simulink model "suspension_controller_road_condition2"  (R2020a)
settings: Solver=VariableStepAuto  StartTime=0.0  StopTime=10.0  MaxStep=0.1  RelTol=1e-3
values from neighbouring files (symbols this model uses):
  cfs = 1290    [half_car_parameter.m]
  cft = 1000    [half_car_parameter.m]
  crs = 1620    [half_car_parameter.m]
  crt = 1000    [half_car_parameter.m]
  iyy = 2460    [half_car_parameter.m]
  kfs = 19960    [half_car_parameter.m]
  kft = 175500    [half_car_parameter.m]
  krs = 17500    [half_car_parameter.m]
  krt = 175500    [half_car_parameter.m]
  lf = 2.3    [half_car_parameter.m]
  lr = 2.3    [half_car_parameter.m]
  mc = 700    [half_car_parameter.m]
  mf = 40    [half_car_parameter.m]
  mr = 35.5    [half_car_parameter.m]
(part 2 of 2)

== system suspension_controller_road_condition2/skyhook/body_sum/sky hook control ==
  zc_dot : Inport
  zc_dot - zf_dot : Inport  Port=2
  Constant : Constant  Value=2838
  Constant1 : Constant  Value=258
  If : If  IfExpression=u1 >= 0  ZeroCross=off
  If Action Subsystem : Subsystem  TreatAsAtomicUnit=on
  If Action Subsystem1 : Subsystem  TreatAsAtomicUnit=on
  Merge : Merge
  Product : Product
  Csa : Outport
  wires:
  zc_dot/1 -> Product/1
  Product/1 -> If/1
  If/1 -> If Action Subsystem/Action
  Constant/1 -> If Action Subsystem/1(In1)
  If/2 -> If Action Subsystem1/Action
  If Action Subsystem/1(Csa) -> Merge/1
  If Action Subsystem1/1(Out1) -> Merge/2
  Merge/1 -> Csa/1
  Constant1/1 -> If Action Subsystem1/1(In1)
  zc_dot - zf_dot/1 -> Product/2

== system suspension_controller_road_condition2/skyhook/body_sum/sky hook control1 ==
  zc_dot : Inport
  zc_dot - zr_dot : Inport  Port=2
  Constant : Constant  Value=2838
  Constant1 : Constant  Value=258
  If : If  IfExpression=u1 >= 0  ZeroCross=off
  If Action Subsystem : Subsystem  TreatAsAtomicUnit=on
  If Action Subsystem1 : Subsystem  TreatAsAtomicUnit=on
  Merge : Merge
  Product : Product
  Csa : Outport
  wires:
  zc_dot/1 -> Product/1
  Product/1 -> If/1
  If/1 -> If Action Subsystem/Action
  Constant/1 -> If Action Subsystem/1(In1)
  If/2 -> If Action Subsystem1/Action
  If Action Subsystem/1(Csa) -> Merge/1
  If Action Subsystem1/1(Out1) -> Merge/2
  Merge/1 -> Csa/1
  Constant1/1 -> If Action Subsystem1/1(In1)
  zc_dot - zr_dot/1 -> Product/2

== system suspension_controller_road_condition2/skyhook/front_sum/Road Condition2 ==
  Product : Product  Inputs=3
  Saturation : Saturate  LowerLimit=0
  Scope : Scope
  Signal Generator : SignalGenerator  Amplitude=0.15  Frequency=1.852
  Step : Step  SampleTime=1.08
  Step1 : Step  Before=1  After=0  SampleTime=4
  Output : Outport
  wires:
  Signal Generator/1 -> Product/1
  Step/1 -> Product/2
  Step1/1 -> Product/3
  Product/1 -> Output/1, Saturation/1
  Saturation/1 -> Scope/1

== system suspension_controller_road_condition2/skyhook/front_sum/sky hook control ==
  zc_dot : Inport
  zc_dot - zf_dot : Inport  Port=2
  Constant : Constant  Value=2838
  Constant1 : Constant  Value=258
  If : If  IfExpression=u1 >= 0  ZeroCross=off
  If Action Subsystem : Subsystem  TreatAsAtomicUnit=on
  If Action Subsystem1 : Subsystem  TreatAsAtomicUnit=on
  Merge : Merge
  Product : Product
  Csa : Outport
  wires:
  zc_dot/1 -> Product/1
  Product/1 -> If/1
  If/1 -> If Action Subsystem/Action
  Constant/1 -> If Action Subsystem/1(In1)
  If/2 -> If Action Subsystem1/Action
  If Action Subsystem/1(Csa) -> Merge/1
  If Action Subsystem1/1(Out1) -> Merge/2
  Merge/1 -> Csa/1
  Constant1/1 -> If Action Subsystem1/1(In1)
  zc_dot - zf_dot/1 -> Product/2

== system suspension_controller_road_condition2/skyhook/rear_sum/Road Condition2 ==
  Product : Product  Inputs=3
  Saturation : Saturate  LowerLimit=0
  Scope : Scope
  Signal Generator : SignalGenerator  Amplitude=0.15  Frequency=1.852
  Step : Step  SampleTime=1.08
  Step1 : Step  Before=1  After=0  SampleTime=4
  Output : Outport
  wires:
  Signal Generator/1 -> Product/1
  Step/1 -> Product/2
  Step1/1 -> Product/3
  Product/1 -> Output/1, Saturation/1
  Saturation/1 -> Scope/1

== system suspension_controller_road_condition2/skyhook/rear_sum/sky hook control ==
  zc_dot : Inport
  zc_dot - zr_dot : Inport  Port=2
  Constant : Constant  Value=2838
  Constant1 : Constant  Value=258
  If : If  IfExpression=u1 >= 0  ZeroCross=off
  If Action Subsystem : Subsystem  TreatAsAtomicUnit=on
  If Action Subsystem1 : Subsystem  TreatAsAtomicUnit=on
  Merge : Merge
  Product : Product
  Csa : Outport
  wires:
  zc_dot/1 -> Product/1
  Product/1 -> If/1
  If/1 -> If Action Subsystem/Action
  Constant/1 -> If Action Subsystem/1(In1)
  If/2 -> If Action Subsystem1/Action
  If Action Subsystem/1(Csa) -> Merge/1
  If Action Subsystem1/1(Out1) -> Merge/2
  Merge/1 -> Csa/1
  Constant1/1 -> If Action Subsystem1/1(In1)
  zc_dot - zr_dot/1 -> Product/2

== system suspension_controller_road_condition2/ground hook/body_sum/Ground hook control/If Action Subsystem ==
  In1 : Inport
  Action Port : ActionPort  ActionPortLabel=if(u1 >= 0)
  Csa : Outport
  wires:
  In1/1 -> Csa/1

== system suspension_controller_road_condition2/ground hook/body_sum/Ground hook control/If Action Subsystem1 ==
  In1 : Inport
  Action Port : ActionPort  ActionPortLabel=else
  Out1 : Outport
  wires:
  In1/1 -> Out1/1

== system suspension_controller_road_condition2/ground hook/body_sum/Ground hook control1/If Action Subsystem ==
  In1 : Inport
  Action Port : ActionPort  ActionPortLabel=if(u1 >= 0)
  Csa : Outport
  wires:
  In1/1 -> Csa/1

== system suspension_controller_road_condition2/ground hook/body_sum/Ground hook control1/If Action Subsystem1 ==
  In1 : Inport
  Action Port : ActionPort  ActionPortLabel=else
  Out1 : Outport
  wires:
  In1/1 -> Out1/1

== system suspension_controller_road_condition2/ground hook/front_sum/Ground hook control/If Action Subsystem ==
  In1 : Inport
  Action Port : ActionPort  ActionPortLabel=if(u1 >= 0)
  Csa : Outport
  wires:
  In1/1 -> Csa/1

== system suspension_controller_road_condition2/ground hook/front_sum/Ground hook control/If Action Subsystem1 ==
  In1 : Inport
  Action Port : ActionPort  ActionPortLabel=else
  Out1 : Outport
  wires:
  In1/1 -> Out1/1

== system suspension_controller_road_condition2/ground hook/rear_sum/Ground hook control1/If Action Subsystem ==
  In1 : Inport
  Action Port : ActionPort  ActionPortLabel=if(u1 >= 0)
  Csa : Outport
  wires:
  In1/1 -> Csa/1

== system suspension_controller_road_condition2/ground hook/rear_sum/Ground hook control1/If Action Subsystem1 ==
  In1 : Inport
  Action Port : ActionPort  ActionPortLabel=else
  Out1 : Outport
  wires:
  In1/1 -> Out1/1

== system suspension_controller_road_condition2/hybrid hook/body_sum/Hybrid controller/If Action Subsystem ==
  In1 : Inport
  Action Port : ActionPort  ActionPortLabel=if(u1 >= 0)
  Csa : Outport
  wires:
  In1/1 -> Csa/1

== system suspension_controller_road_condition2/hybrid hook/body_sum/Hybrid controller/If Action Subsystem1 ==
  In1 : Inport
  Action Port : ActionPort  ActionPortLabel=else
  Out1 : Outport
  wires:
  In1/1 -> Out1/1

== system suspension_controller_road_condition2/hybrid hook/body_sum/Hybrid controller/If Action Subsystem2 ==
  In1 : Inport
  Action Port : ActionPort  ActionPortLabel=if(u1 >= 0)
  Csa : Outport
  wires:
  In1/1 -> Csa/1

== system suspension_controller_road_condition2/hybrid hook/body_sum/Hybrid controller/If Action Subsystem3 ==
  In1 : Inport
  Action Port : ActionPort  ActionPortLabel=else
  Out1 : Outport
  wires:
  In1/1 -> Out1/1

== system suspension_controller_road_condition2/hybrid hook/body_sum/Hybrid controller1/If Action Subsystem ==
  In1 : Inport
  Action Port : ActionPort  ActionPortLabel=if(u1 >= 0)
  Csa : Outport
  wires:
  In1/1 -> Csa/1

== system suspension_controller_road_condition2/hybrid hook/body_sum/Hybrid controller1/If Action Subsystem1 ==
  In1 : Inport
  Action Port : ActionPort  ActionPortLabel=else
  Out1 : Outport
  wires:
  In1/1 -> Out1/1

== system suspension_controller_road_condition2/hybrid hook/body_sum/Hybrid controller1/If Action Subsystem2 ==
  In1 : Inport
  Action Port : ActionPort  ActionPortLabel=if(u1 >= 0)
  Csa : Outport
  wires:
  In1/1 -> Csa/1

== system suspension_controller_road_condition2/hybrid hook/body_sum/Hybrid controller1/If Action Subsystem3 ==
  In1 : Inport
  Action Port : ActionPort  ActionPortLabel=else
  Out1 : Outport
  wires:
  In1/1 -> Out1/1

== system suspension_controller_road_condition2/hybrid hook/front_sum/Hybrid controller/If Action Subsystem ==
  In1 : Inport
  Action Port : ActionPort  ActionPortLabel=if(u1 >= 0)
  Csa : Outport
  wires:
  In1/1 -> Csa/1

== system suspension_controller_road_condition2/hybrid hook/front_sum/Hybrid controller/If Action Subsystem1 ==
  In1 : Inport
  Action Port : ActionPort  ActionPortLabel=else
  Out1 : Outport
  wires:
  In1/1 -> Out1/1

== system suspension_controller_road_condition2/hybrid hook/front_sum/Hybrid controller/If Action Subsystem2 ==
  In1 : Inport
  Action Port : ActionPort  ActionPortLabel=if(u1 >= 0)
  Csa : Outport
  wires:
  In1/1 -> Csa/1

== system suspension_controller_road_condition2/hybrid hook/front_sum/Hybrid controller/If Action Subsystem3 ==
  In1 : Inport
  Action Port : ActionPort  ActionPortLabel=else
  Out1 : Outport
  wires:
  In1/1 -> Out1/1

== system suspension_controller_road_condition2/hybrid hook/rear_sum/Hybrid controller1/If Action Subsystem ==
  In1 : Inport
  Action Port : ActionPort  ActionPortLabel=if(u1 >= 0)
  Csa : Outport
  wires:
  In1/1 -> Csa/1

== system suspension_controller_road_condition2/hybrid hook/rear_sum/Hybrid controller1/If Action Subsystem1 ==
  In1 : Inport
  Action Port : ActionPort  ActionPortLabel=else
  Out1 : Outport
  wires:
  In1/1 -> Out1/1

== system suspension_controller_road_condition2/hybrid hook/rear_sum/Hybrid controller1/If Action Subsystem2 ==
  In1 : Inport
  Action Port : ActionPort  ActionPortLabel=if(u1 >= 0)
  Csa : Outport
  wires:
  In1/1 -> Csa/1

== system suspension_controller_road_condition2/hybrid hook/rear_sum/Hybrid controller1/If Action Subsystem3 ==
  In1 : Inport
  Action Port : ActionPort  ActionPortLabel=else
  Out1 : Outport
  wires:
  In1/1 -> Out1/1

== system suspension_controller_road_condition2/skyhook/body_sum/sky hook control/If Action Subsystem ==
  In1 : Inport
  Action Port : ActionPort  ActionPortLabel=if(u1 >= 0)
  Csa : Outport
  wires:
  In1/1 -> Csa/1

== system suspension_controller_road_condition2/skyhook/body_sum/sky hook control/If Action Subsystem1 ==
  In1 : Inport
  Action Port : ActionPort  ActionPortLabel=else
  Out1 : Outport
  wires:
  In1/1 -> Out1/1

== system suspension_controller_road_condition2/skyhook/body_sum/sky hook control1/If Action Subsystem ==
  In1 : Inport
  Action Port : ActionPort  ActionPortLabel=if(u1 >= 0)
  Csa : Outport
  wires:
  In1/1 -> Csa/1

== system suspension_controller_road_condition2/skyhook/body_sum/sky hook control1/If Action Subsystem1 ==
  In1 : Inport
  Action Port : ActionPort  ActionPortLabel=else
  Out1 : Outport
  wires:
  In1/1 -> Out1/1

== system suspension_controller_road_condition2/skyhook/front_sum/sky hook control/If Action Subsystem ==
  In1 : Inport
  Action Port : ActionPort  ActionPortLabel=if(u1 >= 0)
  Csa : Outport
  wires:
  In1/1 -> Csa/1

== system suspension_controller_road_condition2/skyhook/front_sum/sky hook control/If Action Subsystem1 ==
  In1 : Inport
  Action Port : ActionPort  ActionPortLabel=else
  Out1 : Outport
  wires:
  In1/1 -> Out1/1

== system suspension_controller_road_condition2/skyhook/rear_sum/sky hook control/If Action Subsystem ==
  In1 : Inport
  Action Port : ActionPort  ActionPortLabel=if(u1 >= 0)
  Csa : Outport
  wires:
  In1/1 -> Csa/1

== system suspension_controller_road_condition2/skyhook/rear_sum/sky hook control/If Action Subsystem1 ==
  In1 : Inport
  Action Port : ActionPort  ActionPortLabel=else
  Out1 : Outport
  wires:
  In1/1 -> Out1/1
